simulink model "auto"  (R2021b)
settings: Solver=VariableStepAuto  StartTime=0.0  StopTime=0.1  RelTol=1e-3
libraries: truetime x10
settings Model: Creator=mozzr  LastModifiedBy=mozzr

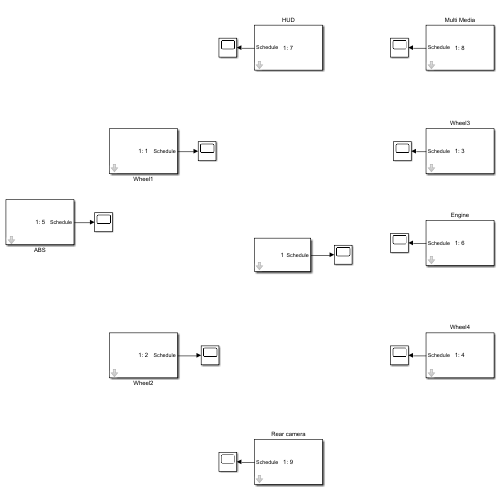
[thumbnail: Simulink's stored preview of the top-level diagram]
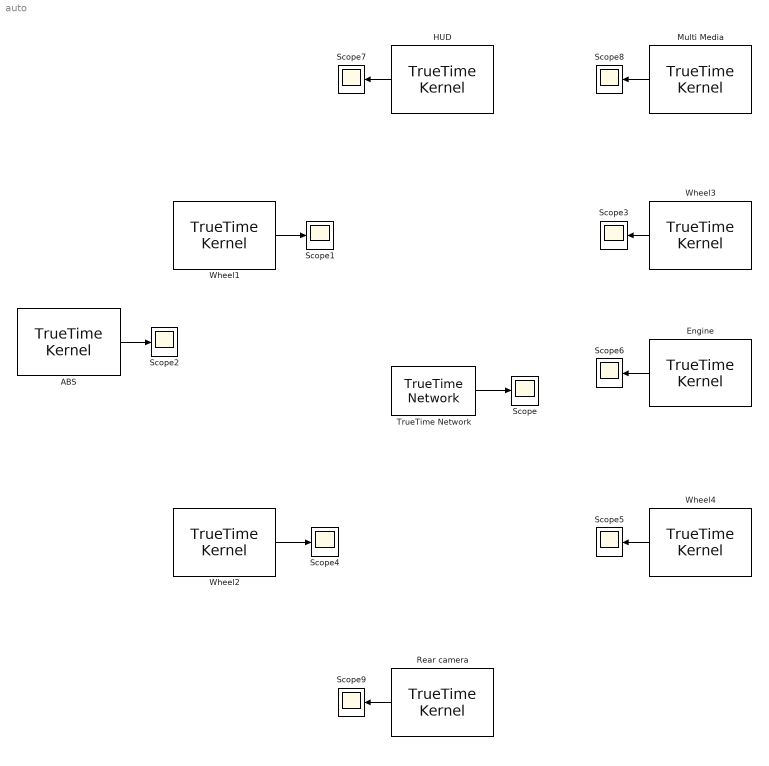
== system auto ==
  ABS : truetime/TrueTime Kernel  sfun=abs_init  args=[]  ninputsoutputs=[0 0]  ntriggers=0  trigtype=falling  nwnodenbr=[1 5]  clockoffsetdrift=[0 0]  schedoutput=on  battery=off  poweroutput=off  label=1: 5
  Engine : truetime/TrueTime Kernel  sfun=engine_init  args=[]  ninputsoutputs=[0 0]  ntriggers=0  trigtype=falling  nwnodenbr=[1 6]  clockoffsetdrift=[0 0]  schedoutput=on  battery=off  poweroutput=off  label=1: 6
  HUD : truetime/TrueTime Kernel  sfun=hud_init  args=[]  ninputsoutputs=[0 0]  ntriggers=0  trigtype=falling  nwnodenbr=[1 7]  clockoffsetdrift=[0 0]  schedoutput=on  battery=off  poweroutput=off  label=1: 7
  Multi Media : truetime/TrueTime Kernel  sfun=media_init  args=[]  ninputsoutputs=[0 0]  ntriggers=0  trigtype=falling  nwnodenbr=[1 8]  clockoffsetdrift=[0 0]  schedoutput=on  battery=off  poweroutput=off  label=1: 8
  Rear camera : truetime/TrueTime Kernel  sfun=camera_init  args=[]  ninputsoutputs=[0 0]  ntriggers=0  trigtype=falling  nwnodenbr=[1 9]  clockoffsetdrift=[0 0]  schedoutput=on  battery=off  poweroutput=off  label=1: 9
  Scope{,1..9} (10 alike) : Scope
  TrueTime Network : truetime/TrueTime Network  nwtype=CSMA/AMP (CAN)  nwnbr=1  nnodes=9  rate=1000000  minsize=1  lossprob=0  seed=0  bandwidths=[0.5 0.5]  slotsize=512  schedule=[1 1 2]  memsize=80000  buftype=Common buffer  overflow=Retransmit  dynSchedule=0  miniSlotSize=0  NIT=0  QSortMode=FIFO  sync=0  irtSchedule=0  nrtLength=0  nodeGraph=0  scheduleoutput=on
  Wheel1 : truetime/TrueTime Kernel  sfun=wheel1_init  args=[]  ninputsoutputs=[0 0]  ntriggers=0  trigtype=falling  nwnodenbr=[1 1]  clockoffsetdrift=[0 0]  schedoutput=on  battery=off  poweroutput=off  label=1: 1
  Wheel2 : truetime/TrueTime Kernel  sfun=wheel2_init  args=[]  ninputsoutputs=[0 0]  ntriggers=0  trigtype=falling  nwnodenbr=[1 2]  clockoffsetdrift=[0 0]  schedoutput=on  battery=off  poweroutput=off  label=1: 2
  Wheel3 : truetime/TrueTime Kernel  sfun=wheel3_init  args=[]  ninputsoutputs=[0 0]  ntriggers=0  trigtype=falling  nwnodenbr=[1 3]  clockoffsetdrift=[0 0]  schedoutput=on  battery=off  poweroutput=off  label=1: 3
  Wheel4 : truetime/TrueTime Kernel  sfun=wheel4_init  args=[]  ninputsoutputs=[0 0]  ntriggers=0  trigtype=falling  nwnodenbr=[1 4]  clockoffsetdrift=[0 0]  schedoutput=on  battery=off  poweroutput=off  label=1: 4
  wires:
  TrueTime Network/1 -> Scope/1
  Wheel1/1 -> Scope1/1
  ABS/1 -> Scope2/1
  Wheel3/1 -> Scope3/1
  Wheel4/1 -> Scope5/1
  Wheel2/1 -> Scope4/1
  Engine/1 -> Scope6/1
  HUD/1 -> Scope7/1
  Multi Media/1 -> Scope8/1
  Rear camera/1 -> Scope9/1
